simulink model "harmonicsTest"  (R2021a)
settings: Solver=FixedStepDiscrete  StartTime=0.0  StopTime=stopTime  RelTol=1e-3
PostLoadFcn:
  | addpath([fileparts(which(bdroot)) filesep '..' filesep])
InitFcn:
  | simulinkInitHarmonics
StopFcn:
  | simulinkVerifyHarmonics
undefined symbols (not defined in the file or in its folder): params
libraries: dspsrcs4 x1
settings Model: DataTypeOverride=Off  SimulationMode=accelerator  PauseTimes=1  Creator=trevor  LastModifiedBy=trevor
settings SolverCC: AlgebraicLoopSolver=TrustRegion
settings DataIOCC: SaveFormat=Array  SaveOutput=off  DSMLogging=off  SaveTime=off  ReturnWorkspaceOutputs=off
settings OptimizationCC: BlockReduction=off  ConditionallyExecuteInputs=off  DefaultParameterBehavior=Inlined
settings DebuggingCC: AlgebraicLoopMsg=error  SingleTaskRateTransMsg=error
settings HardwareCC: ProdBitPerPointer=32  ProdBitPerSizeT=32  ProdBitPerPtrDiffT=32  ProdLargestAtomicFloat=None  ProdIntDivRoundTo=Undefined  ProdEndianess=Unspecified  ProdWordSize=32  ProdHWDeviceType=ASIC/FPGA->ASIC/FPGA  TargetBitPerLong=64  TargetBitPerPointer=64  TargetBitPerSizeT=64  TargetBitPerPtrDiffT=64  TargetLongLongMode=on  TargetIntDivRoundTo=Zero  TargetEndianess=LittleEndian  TargetWordSize=64  TargetHWDeviceType=Custom Processor->MATLAB Host Computer  ProdEqTarget=off

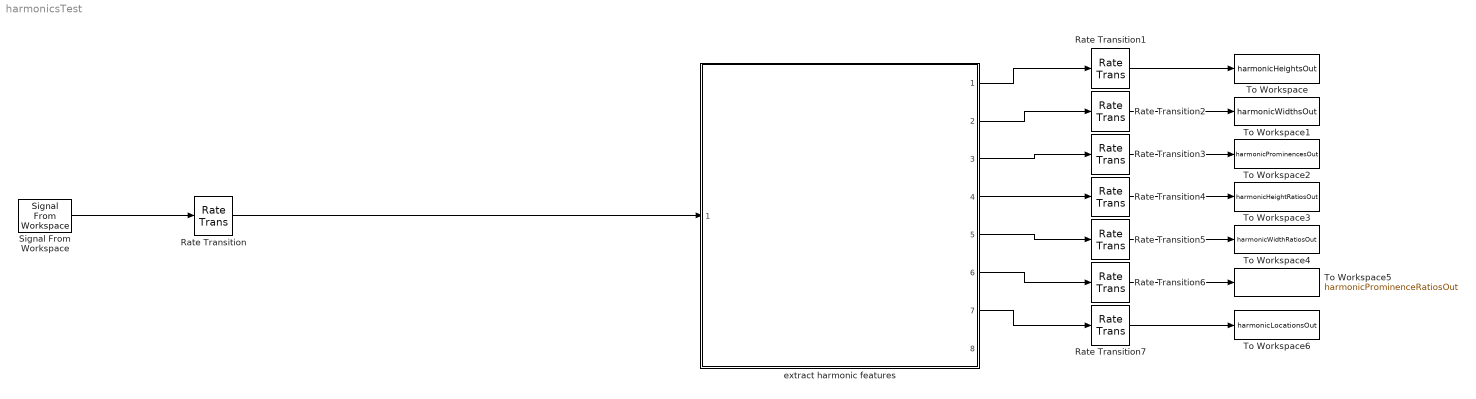
== system harmonicsTest ==
  Rate Transition : RateTransition  Deterministic=off  OutPortSampleTime=params.systemClockPeriod
  Rate Transition{1..7} (7 alike) : RateTransition  OutPortSampleTime=params.samplingPeriod
  Signal From Workspace : dspsrcs4/Signal From Workspace  X=esd  Ts=params.samplingPeriod  nsamps=1  OutputAfterFinalValue=Setting to zero  ignoreOrWarnInputAndFrameLengths=off  OutputFrames=off
  To Workspace : ToWorkspace  VariableName=harmonicHeightsOut  SampleTime=-1
      settings: Save2DSignal=2-D array (concatenate along first dimension)
  To Workspace1 : ToWorkspace  VariableName=harmonicWidthsOut  SampleTime=-1
      settings: Save2DSignal=2-D array (concatenate along first dimension)
  To Workspace2 : ToWorkspace  VariableName=harmonicProminencesOut  SampleTime=-1
      settings: Save2DSignal=2-D array (concatenate along first dimension)
  To Workspace3 : ToWorkspace  VariableName=harmonicHeightRatiosOut  SampleTime=-1
      settings: Save2DSignal=2-D array (concatenate along first dimension)
  To Workspace4 : ToWorkspace  VariableName=harmonicWidthRatiosOut  SampleTime=-1
      settings: Save2DSignal=2-D array (concatenate along first dimension)
  To Workspace5 : ToWorkspace  VariableName=harmonicProminenceRatiosOut  SampleTime=-1
      settings: Save2DSignal=2-D array (concatenate along first dimension)
  To Workspace6 : ToWorkspace  VariableName=harmonicLocationsOut  SampleTime=-1
      settings: Save2DSignal=2-D array (concatenate along first dimension)
  extract harmonic features : Subsystem  ReferencedSubsystem=harmonicFeatures
  wires:
  Signal From Workspace/1 -> Rate Transition/1
  Rate Transition1/1 -> To Workspace/1
  extract harmonic features/1 -> Rate Transition1/1
  Rate Transition2/1 -> To Workspace1/1
  extract harmonic features/2 -> Rate Transition2/1
  Rate Transition3/1 -> To Workspace2/1
  extract harmonic features/3 -> Rate Transition3/1
  extract harmonic features/4 -> Rate Transition4/1
  Rate Transition4/1 -> To Workspace3/1
  extract harmonic features/5 -> Rate Transition5/1
  Rate Transition5/1 -> To Workspace4/1
  extract harmonic features/6 -> Rate Transition6/1
  Rate Transition6/1 -> To Workspace5/1
  extract harmonic features/7 -> Rate Transition7/1
  Rate Transition7/1 -> To Workspace6/1
  Rate Transition/1 -> extract harmonic features/1
